simulink model "complete_model_ol"  (R2020b)
settings: Solver=ode45  StartTime=0  StopTime=8001.99  FixedStep=0.01  RelTol=1e-3
values from neighbouring files (symbols this model uses):
  T_amb = 15    [set_up_parameters_for_simulink.m]
  T_c = 1    [run_benchmark.m]    (also in simulate_OL.m)
  T_sim = 1e-2    (= 0.01)    [set_up_parameters_for_simulink.m]
undefined symbols (not defined in the file or in its folder): possible_ppms, success_rates_packs_temperatures
settings Model: Creator=leop9  LastModifiedBy=Lenyor

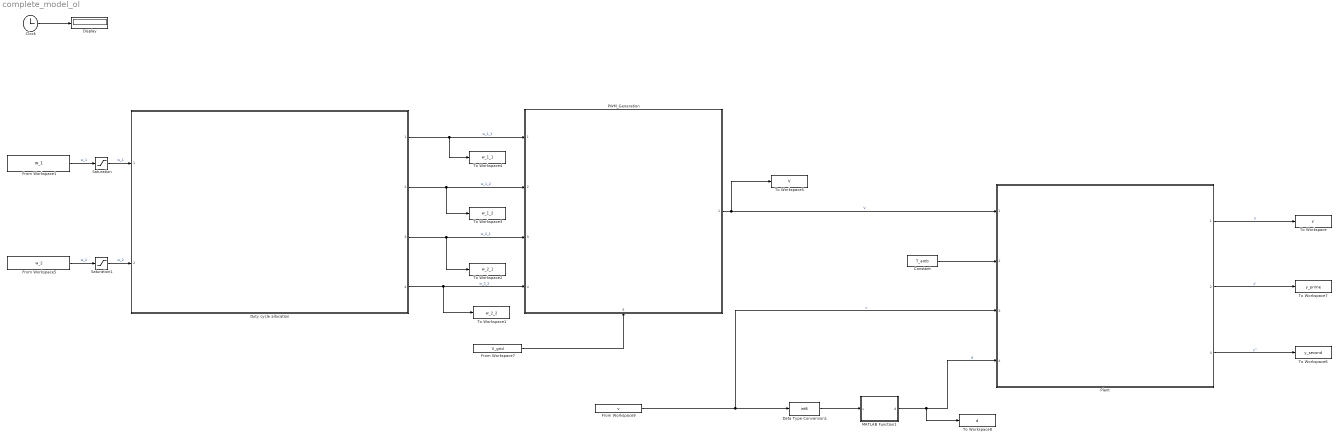
== system complete_model_ol ==
  Clock : Clock
  Constant : Constant  Value=T_amb
  Data Type Conversion1 : DataTypeConversion  OutDataTypeStr=int8
  Display : Display
  Duty cycle allocation : Subsystem  ReferencedSubsystem=duty_cycle_allocation_T_PWM_1
  From Workspace1 : FromWorkspace  VariableName=w_1  SampleTime=T_c
  From Workspace5 : FromWorkspace  VariableName=w_2  SampleTime=T_c
  From Workspace7 : FromWorkspace  VariableName=V_grid  SampleTime=T_sim
  From Workspace9 : FromWorkspace  VariableName=v  SampleTime=T_sim
  MATLAB Function1 : MATLAB Function  TreatAsAtomicUnit=on
  PWM_Generation : Subsystem  ReferencedSubsystem=PWM_generation
      settings: PortSchema="{\"entries\":[{\"content\":{\"sides\":[{\"content\":{\"connectorIds\":[\"In1\",\"In2\",\"In3\",\"In4\"]},\"type\":\"ConnectorPlacement.EquallySpacedRectSide\",\"uuid\":\"fe032f5a-a289-47cb-afea-806cec025375\"},{\"content\":{\"connectorIds\":[\"Out1\"],\"side\":\"RIGHT\"},\"type\":\"ConnectorPlacement.EquallySpacedRectSide\",\"uuid\":\"9e11d798-72c3-41e5-8706-3d056dfacaa8\"},{\"content\":{\"connectorIds\":[],\"side\":\"TOP\"},\"type\":\"ConnectorPlacement.EquallySpacedRectSide\",\"uuid\":\"490c4c10-586f-4d7a-a82e-a8a5f00567fd\"},{\"content\":{\"connectorIds\":[\"In5\"],\"side\":\"BOTTOM\"},\"type\":\"ConnectorPlacement.EquallySpacedRectSide\",\"uuid\":\"f2e91da2-031d-4acf-99af-d2f020191194\"},{\"content\":{\"connectorIds\":[],\"side\":\"HIDDEN\"},\"type\":\"ConnectorPlacement.EquallySpacedRectSide\",\"uuid\":\"b0d0fe5a-b4b0-40c0-ba4b-1f103e92609d\"}]},\"type\":\"ConnectorPlacement.EquallySpacedConnector\",\"uuid\":\"05cf0ac9-0da2-484a-9ea4-a5cb87b84c7e\"}],\"packageUris\":[\"http://schema.mathworks.com/mf0/Connector/R2020b\"],\"version\":\"1.0\"}"
  Plant : Subsystem  ReferencedSubsystem=plant
  Saturation : Saturate  UpperLimit=1  LowerLimit=0
  Saturation1 : Saturate  UpperLimit=1  LowerLimit=0
  To Workspace : ToWorkspace  VariableName=y  SaveFormat=Timeseries  SampleTime=T_sim
  To Workspace1 : ToWorkspace  VariableName=w_2_2  SaveFormat=Timeseries  SampleTime=T_sim
  To Workspace2 : ToWorkspace  VariableName=w_2_1  SaveFormat=Timeseries  SampleTime=T_sim
  To Workspace3 : ToWorkspace  VariableName=w_1_2  SaveFormat=Timeseries  SampleTime=T_sim
  To Workspace4 : ToWorkspace  VariableName=w_1_1  SaveFormat=Timeseries  SampleTime=T_sim
  To Workspace5 : ToWorkspace  VariableName=V  SaveFormat=Timeseries  SampleTime=T_sim
  To Workspace6 : ToWorkspace  VariableName=y_second  SaveFormat=Timeseries  SampleTime=T_sim
  To Workspace7 : ToWorkspace  VariableName=y_prime  SaveFormat=Timeseries  SampleTime=T_sim
  To Workspace8 : ToWorkspace  VariableName=d  SaveFormat=Timeseries  SampleTime=T_sim
  wires:
  Data Type Conversion1/1 -> MATLAB Function1/1(v)
  From Workspace9/1 -> Plant/3, Data Type Conversion1/1  "v"
  Plant/1 -> To Workspace/1  "y"
  From Workspace1/1 -> Saturation/1  "w_1"
  From Workspace5/1 -> Saturation1/1  "w_2"
  From Workspace7/1 -> PWM_Generation/5
  Duty cycle allocation/4 -> PWM_Generation/4, To Workspace1/1  "w_2_2"
  Duty cycle allocation/2 -> To Workspace3/1, PWM_Generation/2  "w_1_2"
  PWM_Generation/1 -> Plant/1, To Workspace5/1  "V"
  Duty cycle allocation/1 -> PWM_Generation/1, To Workspace4/1  "w_1_1"
  Duty cycle allocation/3 -> PWM_Generation/3, To Workspace2/1  "w_2_1"
  Constant/1 -> Plant/2
  MATLAB Function1/1(d) -> To Workspace8/1, Plant/4  "d"
  Plant/2 -> To Workspace7/1  "y'"
  Plant/3 -> To Workspace6/1  "y''"
  Saturation/1 -> Duty cycle allocation/1  "w_1"
  Saturation1/1 -> Duty cycle allocation/2  "w_2"
  Clock/1 -> Display/1

== matlab function complete_model_ol/MATLAB Function1 ==
  data: v input; d output; possible_ppms parameter; success_rates_packs_temperatures parameter
function d = d_generator(v, possible_ppms, success_rates_packs_temperatures)
d = 0;

switch v
    case possible_ppms(1)
        d = pseudo_bernoulli(success_rates_packs_temperatures(1), 1);
    case possible_ppms(2)
        d = pseudo_bernoulli(success_rates_packs_temperatures(2), 1);
    case possible_ppms(3)
        d = pseudo_bernoulli(success_rates_packs_temperatures(3), 1);
    otherwise
        d = 0;
     
end
